simulink model "quartercar"  (R2013a)
settings: Solver=ode45  StartTime=0.0  StopTime=100  RelTol=1e-3
PreLoadFcn:
  | mb=2500;
  | mw=320;
  | k1=80000;
  | k2=500000;
  | b1=320;
  | b2=15020;
settings Model: Creator=Sukriti Singh  LastModifiedBy=Sukriti Singh

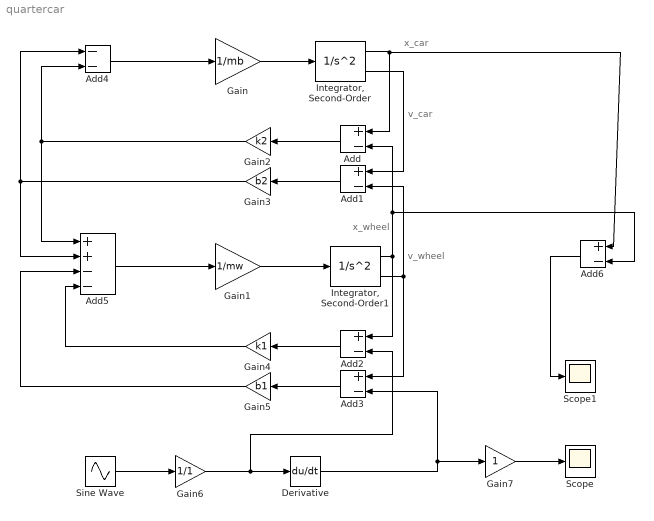
== system quartercar ==
  note: v_wheel
  note: x_wheel
  note: x_car
  note: v_car
  Add{,1..3,6} (5 alike) : Sum  Inputs=+-
  Add4 : Sum  Inputs=--
  Add5 : Sum  Inputs=++--
  Derivative : Derivative
  Gain : Gain  Gain=1/mb
  Gain1 : Gain  Gain=1/mw
  Gain2 : Gain  Gain=k2
  Gain3 : Gain  Gain=b2
  Gain4 : Gain  Gain=k1
  Gain5 : Gain  Gain=b1
  Gain6 : Gain  Gain=1/1
  Gain7 : Gain
  "Integrator, Second-Order" : SecondOrderIntegrator
  "Integrator, Second-Order1" : SecondOrderIntegrator
  Scope : Scope
  Scope1 : Scope
      settings: SaveName=Z
  Sine Wave : Sin  SampleTime=0
  wires:
  Derivative/1 -> Add3/2, Gain7/1
  Add3/1 -> Gain5/1
  Add2/1 -> Gain4/1
  Gain1/1 -> "Integrator, Second-Order1"/1
  Add1/1 -> Gain3/1
  Add/1 -> Gain2/1
  Gain/1 -> "Integrator, Second-Order"/1
  Add4/1 -> Gain/1
  Add5/1 -> Gain1/1
  Gain2/1 -> Add5/1, Add4/2
  Gain3/1 -> Add4/1, Add5/2
  Gain4/1 -> Add5/4
  Gain5/1 -> Add5/3
  "Integrator, Second-Order"/1 -> Add6/1, Add/1
  "Integrator, Second-Order"/2 -> Add1/1
  "Integrator, Second-Order1"/1 -> Add2/1, Add6/2, Add/2
  "Integrator, Second-Order1"/2 -> Add1/2, Add3/1
  Sine Wave/1 -> Gain6/1
  Gain6/1 -> Add2/2, Derivative/1
  Gain7/1 -> Scope/1
  Add6/1 -> Scope1/1
